simulink model "Session_2"  (R2020b)
settings: Solver=VariableStepAuto  StartTime=0.0  StopTime=10.0  RelTol=1e-3
InitFcn:
  | run('Session2.m')
values from neighbouring files (symbols this model uses):
  alpha = 0.2    [Session2.m]
  D1 = randi([0,M-1 ],1,N)    [Session2.m]
  frame = [f22 f11]    [Session2.m]
  header = (-1).^H    [Session2.m]
  hh = numel(H)    [Session2.m]
  L = length(frame)    [Session2.m]
  N = 1e3    (= 1000)    [Session2.m]
  pp = 20    [Session2.m]
  Rs = 1e4    (= 10000)    [Session2.m]
  Span = 10    [Session2.m]
  SPS = 8    [Session2.m]
libraries: commfilt2 x2, simulink x1, commsink2 x1, commdigbbndpm3 x1, commchan3 x1
settings Model: Creator=ali hosseini  LastModifiedBy=ali hosseini

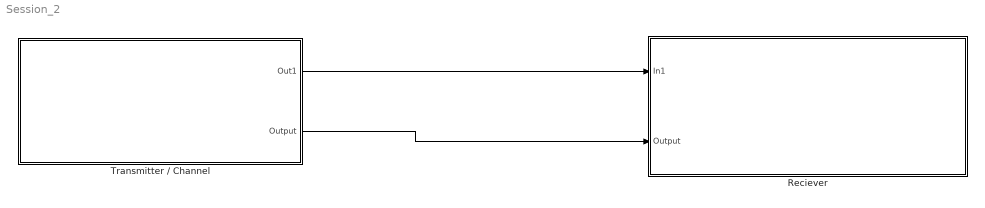
== system Session_2 ==
  Reciever : Subsystem
  Transmitter / Channel : Subsystem
  wires:
  Transmitter / Channel/1(Out1) -> Reciever/1(In1)
  Transmitter / Channel/2(Output) -> Reciever/2(Output)

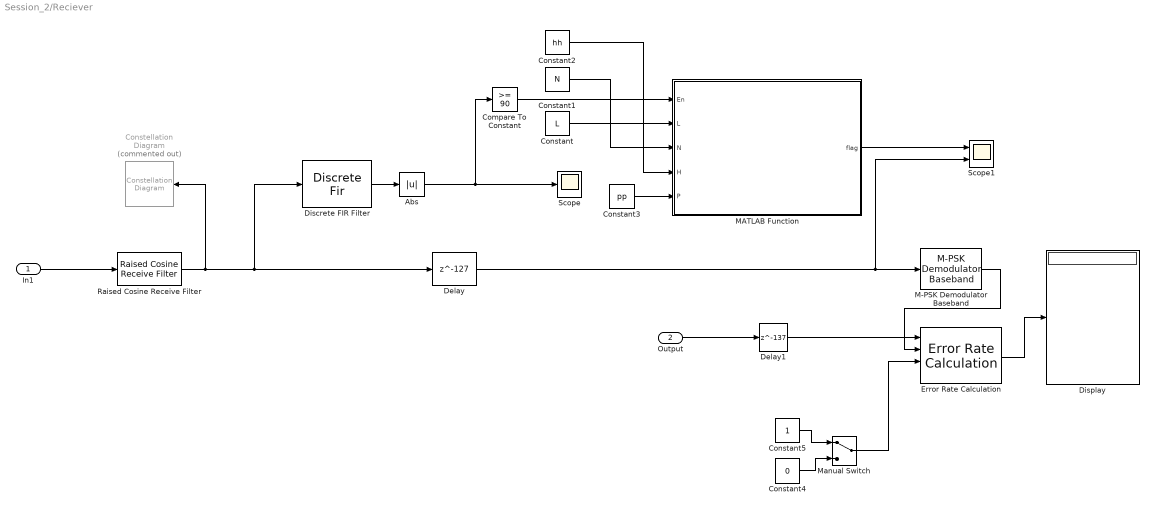
== system Session_2/Reciever ==
  In1 : Inport
  Output : Inport  Port=2
  Abs : Abs
  Compare To Constant : simulink/Logic and Bit Operations/Compare To Constant  relop=>=  const=90  OutDataTypeStr=boolean
  Constant : Constant  Value=L  SampleTime=1/Rs
  Constant1 : Constant  Value=N  SampleTime=1/Rs
  Constant2 : Constant  Value=hh  SampleTime=1/Rs
  Constant3 : Constant  Value=pp  SampleTime=1/Rs
  Constant4 : Constant  Value=0
  Constant5 : Constant
  Constellation Diagram : ConstellationDiagram  Commented=on
  Delay : Delay  DelayLength=127  InputProcessing=Columns as channels (frame based)
  Delay1 : Delay  DelayLength=137
  Discrete FIR Filter : DiscreteFir  Coefficients=fliplr(header)
  Display : Display
  Error Rate Calculation : commsink2/Error Rate Calculation  N=0  st_delay=0  cp_mode=Select samples from port  subframe=[]  PMode=Port  WsName=ErrorVec  RsMode2=on  stop=off  numErr=100  maxBits=1e6
  M-PSK Demodulator Baseband : commdigbbndpm3/M-PSK Demodulator Baseband  M=M  OutType=Integer  DecType=Hard decision  VarSource=Dialog  Variance=1  Dec=Gray  Mapping=[0:7]  Ph=pi/M - (pi/M)*(M ==2)  outDtype1=Inherit via internal rule  outDtype2=Inherit via internal rule  derotateFactorWordLen=16  derotateFactorDataTypeStr=Inherit: Same word length as input  derotateFactorLastDataTypeStr=Inherit: Same word length as input
  MATLAB Function : MATLAB Function  TreatAsAtomicUnit=on
  Manual Switch : ManualSwitch
  Raised Cosine Receive Filter : commfilt2/Raised Cosine Receive Filter  filtType=Square root  R=alpha  filtSpan=Span  N=SPS  downFactor=SPS  downOffset=0  filterGain=1  InputProcessing=Columns as channels (frame based)  RateOptions=Allow multirate processing  framing=Mute  checkCoeff=off  variableName=rcRxFilt  currentFiltSpan=Span  D=(Span)/2  inputOffset=0  sampMode=Mute  saveAsFlag=0  rateMode=Downsampling  checkGain=Normalized  launchFVT=on  roundingMode=Floor  overflowMode=off  coeffDataTypeStr=Inherit: Same word length as input  coeffMin=[]  coeffMax=[]  coeffLastDataTypeStr=Inherit: Same word length as input  accumDataTypeStr=Inherit: Same as product output  accumLastDataTypeStr=Inherit: Same as product output  outputDataTypeStr=Inherit: Same as accumulator  outputMin=[]  outputMax=[]  outputLastDataTypeStr=Inherit: Same as accumulator
  Scope : Scope
  Scope1 : Scope  NumInputPorts=2
  wires:
  In1/1 -> Raised Cosine Receive Filter/1
  Raised Cosine Receive Filter/1 -> Constellation Diagram/1, Delay/1, Discrete FIR Filter/1
  Discrete FIR Filter/1 -> Abs/1
  Abs/1 -> Compare To Constant/1, Scope/1
  Compare To Constant/1 -> MATLAB Function/1(En)
  Constant/1 -> MATLAB Function/2(L)
  Constant1/1 -> MATLAB Function/3(N)
  Constant2/1 -> MATLAB Function/4(H)
  Constant3/1 -> MATLAB Function/5(P)
  MATLAB Function/1(flag) -> Scope1/1
  Delay/1 -> M-PSK Demodulator Baseband/1, Scope1/2
  Error Rate Calculation/1 -> Display/1
  Constant4/1 -> Manual Switch/2
  Constant5/1 -> Manual Switch/1
  Manual Switch/1 -> Error Rate Calculation/3
  M-PSK Demodulator Baseband/1 -> Error Rate Calculation/2
  Delay1/1 -> Error Rate Calculation/1
  Output/1 -> Delay1/1

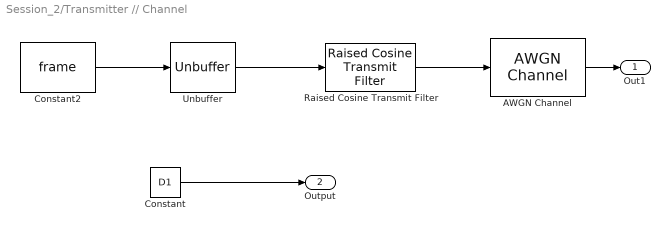
== system Session_2/Transmitter // Channel ==
  AWGN Channel : commchan3/AWGN Channel  InputProcessing=Columns as channels (frame based)  seed=67  noiseMode="Signal to noise ratio  (SNR)"  EbNodB=10  EsNodB=10  SNRdB=30  bitsPerSym=1  Ps=1/SPS  Tsym=1/Rs  variance=1
  Constant : Constant  Value=D1
  Constant2 : Constant  Value=frame  SampleTime=L/Rs  LockScale=on
  Raised Cosine Transmit Filter : commfilt2/Raised Cosine Transmit Filter  filtType=Square root  R=alpha  filtSpan=Span  N=SPS  filterGain=1  InputProcessing=Columns as channels (frame based)  RateOptions=Allow multirate processing  framing=Mute  checkCoeff=off  variableName=rcTxFilt  checkGain=Normalized  sampMode=Mute  saveAsFlag=0  currentFiltSpan=Span  D=(Span)/2  launchFVT=on  roundingMode=Floor  overflowMode=off  coeffDataTypeStr=Inherit: Same word length as input  coeffMin=[]  coeffMax=[]  coeffLastDataTypeStr=Inherit: Same word length as input  outputDataTypeStr=Inherit: Same as accumulator  outputMin=[]  outputMax=[]  outputLastDataTypeStr=Inherit: Same as accumulator
  Unbuffer : Unbuffer
  Out1 : Outport
  Output : Outport  Port=2
  wires:
  Unbuffer/1 -> Raised Cosine Transmit Filter/1
  Constant2/1 -> Unbuffer/1
  Raised Cosine Transmit Filter/1 -> AWGN Channel/1
  AWGN Channel/1 -> Out1/1
  Constant/1 -> Output/1

== matlab function Session_2/Reciever/MATLAB Function ==
  data: En input; flag output; L input; N input; H input; P input
function flag = flagDet(En,L,N,H,P)
    persistent n ;
    if isempty(n)
        n = 0;
    end
    
    flag = 3; %Data 
    if n < H
        flag = 1 ; %header
    elseif  ( n >= H + N && n < H + N +  P) || ( n >= H + 2*N + P && n < 2*P + 2*N + H)
        flag = 2; %flag 
    end
    
    if En
        n = 0 ;
    end
    n = mod(n + 1 , L);
end
